simulink model "model_3_2"  (R2018b)
settings: Solver=VariableStepAuto  StartTime=0.0  StopTime=Endtime  RelTol=1e-3
values from neighbouring files (symbols this model uses):
  D1 = 1 * 10^(-2)    (= 0.01)    [sim_3__2.m]
  D2 = 2 * 10^(-2)    (= 0.02)    [sim_3__2.m]
  J1 = 1 * 10^(-2)    (= 0.01)    [sim_3__2.m]
  J2 = 2 * 10^(-2)    (= 0.02)    [sim_3__2.m]
  K = 1 * 10^(-1)    (= 0.1)    [sim_3__2.m]
  smp = 0.01    [sim_3__2.m]
  tau1 = 1    [sim_3__2.m]
  tau2 = -1    [sim_3__2.m]
settings Model: Creator=nharada  LastModifiedBy=nharada

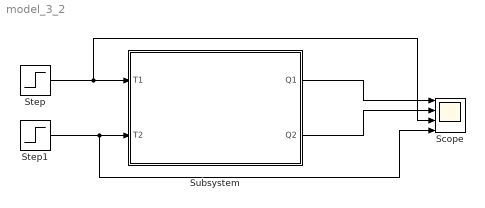
== system model_3_2 ==
  Scope : Scope  NumInputPorts=4
  Step : Step  After=tau1  SampleTime=smp
  Step1 : Step  Time=15  After=tau2  SampleTime=smp
  Subsystem : Subsystem
  wires:
  Step/1 -> Scope/3, Subsystem/1(T1)
  Step1/1 -> Scope/4, Subsystem/2(T2)
  Subsystem/1(Q1) -> Scope/1
  Subsystem/2(Q2) -> Scope/2

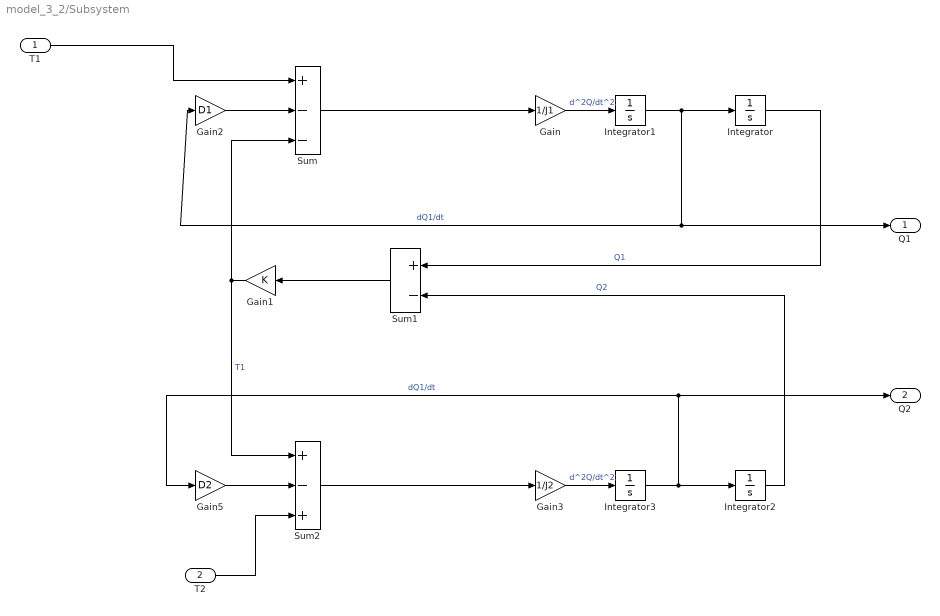
== system model_3_2/Subsystem ==
  T1 : Inport
  T2 : Inport  Port=2
  Gain : Gain  Gain=1/J1
  Gain1 : Gain  Gain=K
  Gain2 : Gain  Gain=D1
  Gain3 : Gain  Gain=1/J2
  Gain5 : Gain  Gain=D2
  Integrator{,1..3} (4 alike) : Integrator
  Sum : Sum  Inputs=+--
  Sum1 : Sum  Inputs=+-
  Sum2 : Sum  Inputs=+-+
  Q1 : Outport
  Q2 : Outport  Port=2
  wires:
  Gain/1 -> Integrator1/1  "d^2Q/dt^2"
  T2/1 -> Sum2/3
  Integrator1/1 -> Q1/1, Gain2/1, Integrator/1  "dQ1/dt"
  Gain2/1 -> Sum/2
  Gain1/1 -> Sum2/1, Sum/3  "T1"
  Integrator2/1 -> Sum1/2  "Q2"
  Integrator3/1 -> Integrator2/1, Gain5/1, Q2/1  "dQ1/dt"
  Integrator/1 -> Sum1/1  "Q1"
  Gain5/1 -> Sum2/2
  Sum/1 -> Gain/1
  T1/1 -> Sum/1
  Sum2/1 -> Gain3/1
  Sum1/1 -> Gain1/1
  Gain3/1 -> Integrator3/1  "d^2Q/dt^2"
